simulink model "TestFlightSim1D"  (R2020b)
settings: Solver=VariableStepAuto  StartTime=0.0  StopTime=80  RelTol=1e-10
settings Model: Creator=jonathan  LastModifiedBy=jonathan

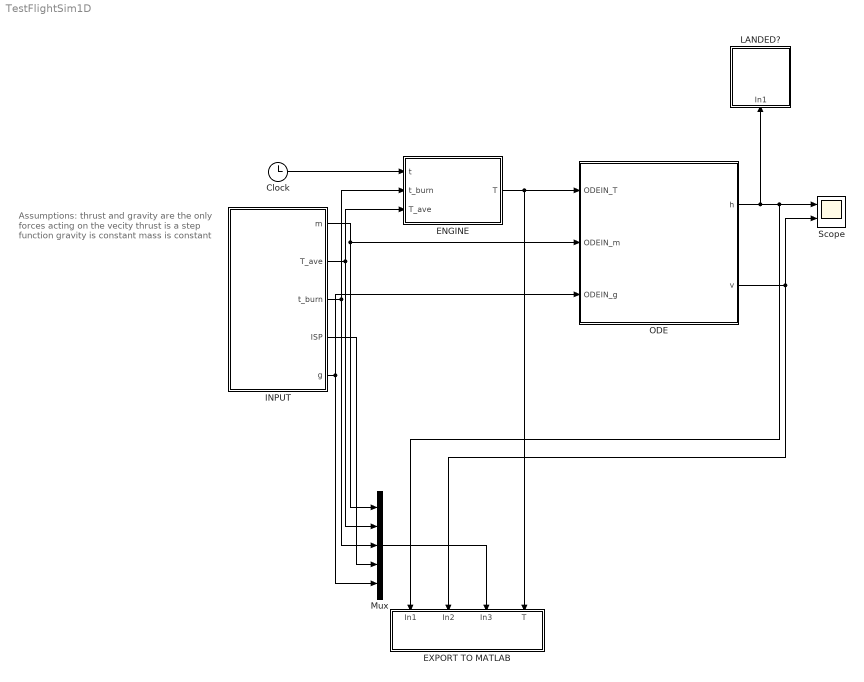
== system TestFlightSim1D ==
  note: Assumptions:
      | thrust and gravity are the only forces acting on the vecity
      | thrust is a step function
      | gravity is constant
      | mass is constant
  Clock : Clock
  ENGINE : MATLAB Function  TreatAsAtomicUnit=on
  EXPORT TO MATLAB : Subsystem
  INPUT : MATLAB Function  TreatAsAtomicUnit=on
  LANDED? : Subsystem
  Mux : Mux  Inputs=5
  ODE : Subsystem
  Scope : Scope  NumInputPorts=2
  wires:
  Clock/1 -> ENGINE/1(t)
  INPUT/2(T_ave) -> Mux/2, ENGINE/3(T_ave)
  INPUT/3(t_burn) -> Mux/3, ENGINE/2(t_burn)
  INPUT/1(m) -> Mux/1, ODE/2(ODEIN_m)
  INPUT/5(g) -> Mux/5, ODE/3(ODEIN_g)
  ODE/2(v) -> EXPORT TO MATLAB/2(In2), Scope/2
  ODE/1(h) -> EXPORT TO MATLAB/1(In1), Scope/1, LANDED?/1(In1)
  INPUT/4(ISP) -> Mux/4
  Mux/1 -> EXPORT TO MATLAB/3(In3)
  ENGINE/1(T) -> ODE/1(ODEIN_T), EXPORT TO MATLAB/4(T)

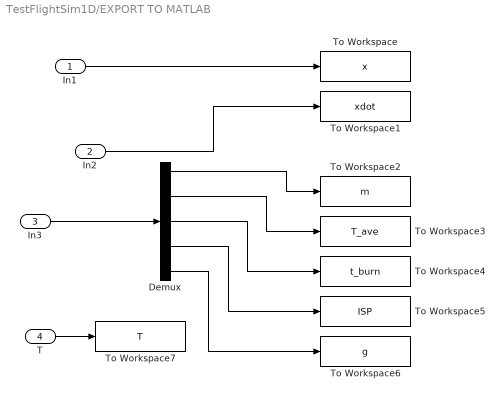
== system TestFlightSim1D/EXPORT TO MATLAB ==
  In1 : Inport
  In2 : Inport  Port=2
  In3 : Inport  Port=3
  T : Inport  Port=4
  Demux : Demux  Outputs=5
  To Workspace : ToWorkspace  VariableName=x  SaveFormat=Timeseries  SampleTime=-1
  To Workspace1 : ToWorkspace  VariableName=xdot  SaveFormat=Timeseries  SampleTime=-1
  To Workspace2 : ToWorkspace  VariableName=m  SaveFormat=Timeseries  SampleTime=-1
  To Workspace3 : ToWorkspace  VariableName=T_ave  SaveFormat=Timeseries  SampleTime=-1
  To Workspace4 : ToWorkspace  VariableName=t_burn  SaveFormat=Timeseries  SampleTime=-1
  To Workspace5 : ToWorkspace  VariableName=ISP  SaveFormat=Timeseries  SampleTime=-1
  To Workspace6 : ToWorkspace  VariableName=g  SaveFormat=Timeseries  SampleTime=-1
  To Workspace7 : ToWorkspace  VariableName=T  SaveFormat=Timeseries  SampleTime=-1
  wires:
  In3/1 -> Demux/1
  In1/1 -> To Workspace/1
  Demux/2 -> To Workspace3/1
  Demux/4 -> To Workspace5/1
  Demux/3 -> To Workspace4/1
  Demux/1 -> To Workspace2/1
  In2/1 -> To Workspace1/1
  Demux/5 -> To Workspace6/1
  T/1 -> To Workspace7/1

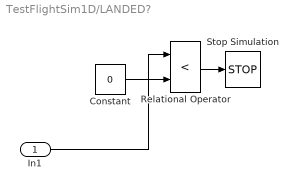
== system TestFlightSim1D/LANDED? ==
  In1 : Inport
  Constant : Constant  Value=0
  Relational Operator : RelationalOperator  Operator=<  OutDataTypeStr=boolean  RndMeth=Simplest
  Stop Simulation : Stop
  wires:
  In1/1 -> Relational Operator/1
  Constant/1 -> Relational Operator/2
  Relational Operator/1 -> Stop Simulation/1

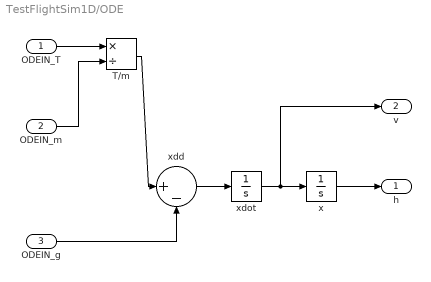
== system TestFlightSim1D/ODE ==
  ODEIN_T : Inport
  ODEIN_m : Inport  Port=2
  ODEIN_g : Inport  Port=3
  T/m : Product  Inputs=*/
  x : Integrator
  xdd : Sum  Inputs=|+-
  xdot : Integrator
  h : Outport
  v : Outport  Port=2
  wires:
  ODEIN_m/1 -> T/m/2
  ODEIN_g/1 -> xdd/2
  ODEIN_T/1 -> T/m/1
  x/1 -> h/1
  xdot/1 -> v/1, x/1
  T/m/1 -> xdd/1
  xdd/1 -> xdot/1

== matlab function TestFlightSim1D/ENGINE ==
  data: t input; t_burn input; T output; T_ave input
function T = fcn(t,t_burn,T_ave)
if t < t_burn
    T = T_ave;
else
    T = 0;
end
end

== matlab function TestFlightSim1D/INPUT ==
  data: m output; T_ave output; t_burn output; ISP output; g output
function [m,T_ave,t_burn,ISP,g] = fcn()
% m - vehicle mass (assumed constant)
% m_fuel - fuel mass
% T_ave - average thrust
% t_burn - burn time
% g - gravitational acceleration (assumed constant)

m = 90; % [kg]
m_fuel = 16; % [kg]
T_ave = 3900; % [N]
ISP = 230; % [kg]
g = 9.8; % [m/s2]

% calculate burntime
t_burn = ISP*9.8*m_fuel/T_ave;

end
